simulink model "CV_Matbab_Moteur"  (R2016a)
settings: Solver=FixedStepAuto  StartTime=0.0  StopTime=10  FixedStep=1e-6  RelTol=1e-3
libraries: powerlib x11
settings Model: SimulationMode=accelerator  Creator=SINA  LastModifiedBy=SINA

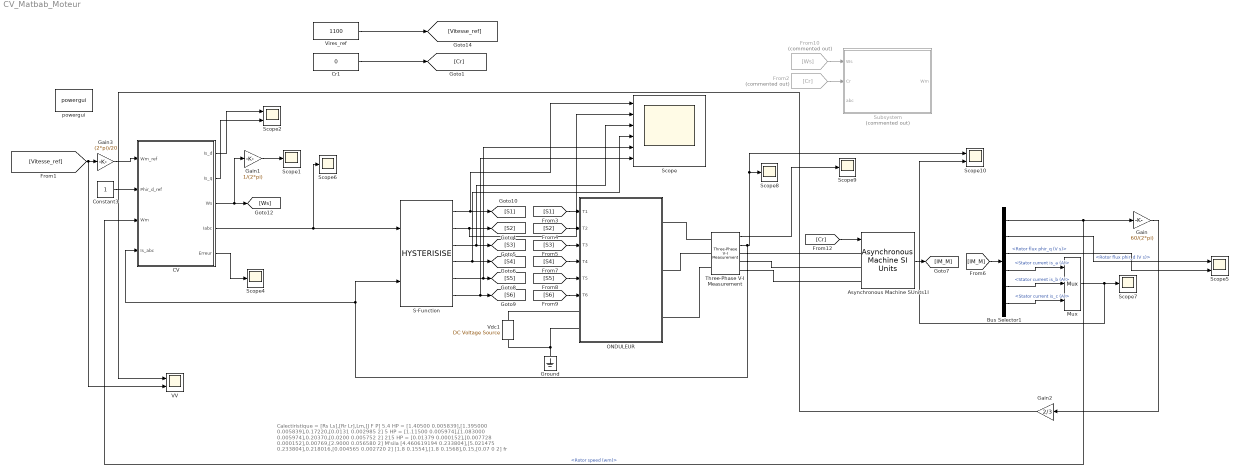
== system CV_Matbab_Moteur ==
  note: Calectiristique = [Rs Ls],[Rr Lr],Lm,[J F P]
      |
      | 5.4 HP = [1.40500 0.005839],[1.395000 0.005839],0.17220,[0.0131 0.002985 2]
      | 5 HP = [1.11500 0.005974],[1.083000 0.005974],0.20370,[0.0200 0.005752 2]
      | 215 HP = [0.01379 0.000152],[0.007728 0.000152],0.00769,[2.9000 0.056580 2]
      |
      | M'sila
      | [4.460619194 0.233804],[5.021475 0.233804],0.218016,[0.004565 0.002720 2]
      |
      | [1.8 0.1554],[1.8 0.1568],0.15,[0.07 0 2] fr
  "Asynchronous Machine SUnits1I " : powerlib/Machines/Asynchronous Machine SI Units  RotorType=Squirrel-cage  PresetModel="15:  5.4 HP (4KW)   400 V  50Hz 1430 RPM"  MechanicalLoad=Torque Tm  ShowDetailedParameters=on  ReferenceFrame=Rotor  Units=SI  MeasurementBus=off  NominalParameters=[4000 400 50]  Stator=[1.405 0.005839]  Rotor=[1.395 0.005839]  Cage1=[0.4155 0.002066]  Cage2=[0.4168 0.0003495]  Lm=0.1722  Mechanical=[0.0131 0.002985 2]  PolePairs=2  InitialConditions=[0 0 0 0 0 0 0 0]  SimulateSaturation=off  Saturation=[14.03593122, 27.81365428, 53.79336849, 72.68890987, 97.98006896, 148.6815601, 215.7428561, 302.9841135, 428.7778367 ; 230, 322, 414, 460, 506, 552, 598, 644, 690]  LoadFlowParameters=1492000  TsPowergui=0  TsBlock=-1  IterativeModel=Trapezoidal non iterative  IterativeDiscreteModel=Trapezoidal non iterative  Pmec=1.492e+006
  Bus Selector1 : BusSelector  OutputSignals=Mechanical.Rotor speed (wm),Rotor measurements.Rotor flux phir_d (V s),Rotor measurements.Rotor flux phir_q (V s),Stator measurements.Stator current is_a (A),Stator measurements.Stator current is_b (A),Stator measurements.Stator current is_c (A)
  CV : Subsystem
  Constant3 : Constant
  Cr1 : Constant  Value=0
  From10 : From  Commented=on  GotoTag=Ws
  From2 : From  Commented=on  GotoTag=Cr
  Gain : Gain  Gain=60/(2*pi)
  Gain1 : Gain  Gain=1/(2*pi)
  Gain2 : Gain  Gain=2/3
  Gain3 : Gain  Gain=(2*pi)/20
  Ground : powerlib/Elements/Ground  LConnTagsString=a
  Mux : Mux  Inputs=3
  ONDULEUR : Subsystem
  S-Function : S-Function  FunctionName=HYSTERISISE  SFunctionDeploymentMode=off  EnableBusSupport=off
  Scope : Scope  NumInputPorts=6
  Scope{1,4,6..9} (6 alike) : Scope
  Scope10 : Scope  NumInputPorts=2
  Scope2 : Scope  NumInputPorts=2
  Scope5 : Scope  NumInputPorts=2
  Subsystem : Subsystem  Commented=on
  Three-Phase V-I Measurement : powerlib/Measurements/Three-Phase V-I Measurement  VoltageMeasurement=phase-to-phase  SetLabelV=off  LabelV=Vabc  Vpu=off  VpuLL=off  CurrentMeasurement=yes  SetLabelI=off  LabelI=Iabc  Ipu=off  Pbase=100e6  Vbase=500e3  OutputType=Complex  PhasorSimulation=off  PSBequivalent=0
  VV : Scope  NumInputPorts=2
  Vdc1 : powerlib/Electrical Sources/DC Voltage Source  Amplitude=650  Measurements=Voltage
  Vires_ref : Constant  Value=1100
  powergui : powerlib/powergui  Priority=1  SimulationMode=Discrete  SolverType=Tustin/Backward Euler (TBE)  SampleTime=1e-6  frequency=60  SPID=off  DisableSnubberDevices=off  DisableRonSwitches=off  DisableVfSwitches=off  SwTol=0  DisplayEquations=off  Interpol=off  ExternalGateDelay=off  methode=off  Ts=0  FunctionMessages=off  echomessages=off  HookPort=off  EnableUseOfTLC=off  x0status=blocks  frequencyindice=0  Pbase=100e6  ErrMax=1e-4  Iterations=50  UnitsV=kV  UnitsW=MW  buscounter=0  RestoreLinks=warning  ResistiveCurrentMeasurement=off  Frange=[0:2:500]  Ylog=off  Xlog=on  ShowGrid=off  save=off  variable=ZData  structure=0  ZoomFFT=on  StartTime=0.0  cycles=1  DisplayStyle=1  fundamental=60  FreqAxis=off  MaxFrequency=1000  frequencyindicesteady=1  RmsSteady=1  display=off
  wires:
  Constant3/1 -> CV/2(Phir_d_ref)
  CV/3(Ws) -> [Ws], Gain1/1
  CV/4(Iabc) -> Scope6/1, S-Function/1
  Gain1/1 -> Scope1/1
  CV/1(Is_d) -> Scope2/1
  CV/2(Is_q) -> Scope2/2
  CV/5(Erreur) -> Scope4/1
  Cr1/1 -> [Cr]
  Vires_ref/1 -> [Vitesse_ref]
  From10/1 -> Subsystem/1(Ws)
  From2/1 -> Subsystem/2(Cr)
  [IM_M] -> Bus Selector1/1
  Bus Selector1/1 -> CV/3(Wm), Gain/1  "<Rotor speed (wm)>"
  "Asynchronous Machine SUnits1I "/1 -> [IM_M]
  [Cr] -> "Asynchronous Machine SUnits1I "/1
  Bus Selector1/2 -> Scope5/1  "<Rotor flux phir_d (V s)>"
  Bus Selector1/3 -> Scope5/2  "<Rotor flux phir_q (V s)>"
  [S1] -> ONDULEUR/1("T1 ")
  [S3] -> ONDULEUR/3("T3  ")
  [S5] -> ONDULEUR/5("T5 ")
  [S2] -> ONDULEUR/2("T2 ")
  [S4] -> ONDULEUR/4("T4 ")
  [S6] -> ONDULEUR/6("T6 ")
  S-Function/5 -> Scope/5, [S5]
  S-Function/4 -> Scope/4, [S4]
  S-Function/3 -> Scope/3, [S3]
  S-Function/2 -> Scope/2, [S2]
  S-Function/1 -> Scope/1, [S1]
  Bus Selector1/4 -> Mux/1  "<Stator current is_a (A)>"
  Bus Selector1/5 -> Mux/2  "<Stator current is_b (A)>"
  Bus Selector1/6 -> Mux/3  "<Stator current is_c (A)>"
  Mux/1 -> Scope10/2, Scope7/1
  S-Function/6 -> Scope/6, [S6]
  Three-Phase V-I Measurement/2 -> S-Function/2, CV/4(Is_abc), Scope10/1, Scope8/1
  Three-Phase V-I Measurement/1 -> Scope9/1
  [Vitesse_ref] -> VV/2, Gain3/1
  Gain3/1 -> CV/1(Wm_ref)
  Gain/1 -> Gain2/1
  Gain2/1 -> VV/1
  connections:
  Three-Phase V-I Measurement/LConn3 -- ONDULEUR/RConn3
  Three-Phase V-I Measurement/LConn2 -- ONDULEUR/RConn2
  Three-Phase V-I Measurement/LConn1 -- ONDULEUR/RConn1
  Three-Phase V-I Measurement/RConn1 -- "Asynchronous Machine SUnits1I "/LConn1
  Three-Phase V-I Measurement/RConn2 -- "Asynchronous Machine SUnits1I "/LConn2
  Three-Phase V-I Measurement/RConn3 -- "Asynchronous Machine SUnits1I "/LConn3
  Vdc1/RConn1 -- ONDULEUR/LConn1
  Ground/LConn1 -- ONDULEUR/LConn2 -- Vdc1/LConn1

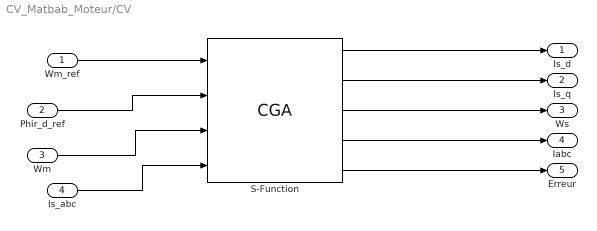
== system CV_Matbab_Moteur/CV ==
  Wm_ref : Inport
  Phir_d_ref : Inport  Port=2
  Wm : Inport  Port=3
  Is_abc : Inport  Port=4
  S-Function : S-Function  FunctionName=CGA  Parameters=[1.40500 0.005839],[1.395000 0.005839],0.17220,[0.0131 0.002985 2]  SFunctionDeploymentMode=off  EnableBusSupport=off
  Is_d : Outport
  Is_q : Outport  Port=2
  Ws : Outport  Port=3
  Iabc : Outport  Port=4
  Erreur : Outport  Port=5
  wires:
  S-Function/4 -> Iabc/1
  S-Function/3 -> Ws/1
  S-Function/2 -> Is_q/1
  S-Function/1 -> Is_d/1
  Wm/1 -> S-Function/3
  Phir_d_ref/1 -> S-Function/2
  Wm_ref/1 -> S-Function/1
  S-Function/5 -> Erreur/1
  Is_abc/1 -> S-Function/4

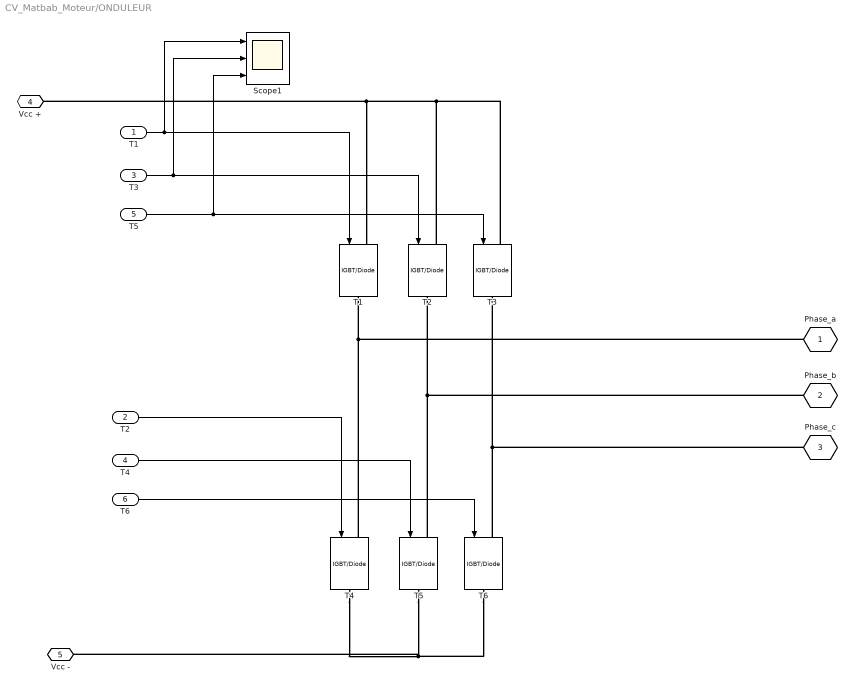
== system CV_Matbab_Moteur/ONDULEUR ==
  "T1 " : Inport
  "T2 " : Inport  Port=2
  "T3  " : Inport  Port=3
  "T4 " : Inport  Port=4
  "T5 " : Inport  Port=5
  "T6 " : Inport  Port=6
  Scope1 : Scope  NumInputPorts=3
  T{1..6} (6 alike) : powerlib/Power Electronics/IGBT//Diode  Ron=1e-3  Rs=1e5  Cs=inf  Measurements=off
  Phase_a : PMIOPort  Tag=PMCPort  Port=1  Side=Right
  Phase_b : PMIOPort  Tag=PMCPort  Port=2  Side=Right
  Phase_c : PMIOPort  Tag=PMCPort  Port=3  Side=Right
  Vcc + : PMIOPort  Port=4  Side=Left
  Vcc - : PMIOPort  Port=5  Side=Left
  wires:
  "T1 "/1 -> Scope1/1, T1/1
  "T3  "/1 -> Scope1/2, T2/1
  "T5 "/1 -> Scope1/3, T3/1
  "T2 "/1 -> T4/1
  "T4 "/1 -> T5/1
  "T6 "/1 -> T6/1
  connections:
  T2/LConn1 -- T3/LConn1 -- Vcc +/RConn1 -- T1/LConn1
  T5/RConn1 -- T4/RConn1 -- Vcc -/RConn1 -- T6/RConn1
  T4/LConn1 -- Phase_a/RConn1 -- T1/RConn1
  T5/LConn1 -- Phase_b/RConn1 -- T2/RConn1
  T6/LConn1 -- Phase_c/RConn1 -- T3/RConn1

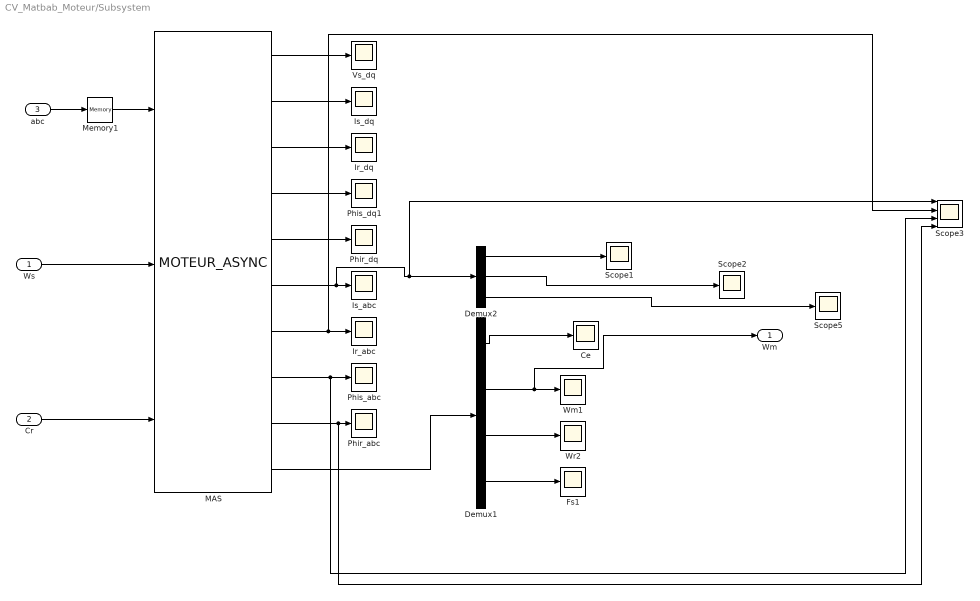
== system CV_Matbab_Moteur/Subsystem ==
  Ws : Inport
  Cr : Inport  Port=2
  abc : Inport  Port=3
  Ce : Scope
  Demux1 : Demux
  Demux2 : Demux  Outputs=3
  Fs1 : Scope
  Ir_abc : Scope
  Ir_dq : Scope
  Is_abc : Scope
  Is_dq : Scope
  MAS : S-Function  FunctionName=MOTEUR_ASYNC  Parameters=[1.40500 0.005839],[1.395000 0.005839],0.17220,[0.0131 0.002985 2]  SFunctionDeploymentMode=off  EnableBusSupport=off
  Memory1 : Memory
  Phir_abc : Scope
  Phir_dq : Scope
  Phis_abc : Scope
  Phis_dq1 : Scope
  Scope1 : Scope
  Scope2 : Scope
  Scope3 : Scope  NumInputPorts=4
  Scope5 : Scope
  Vs_dq : Scope
  Wm1 : Scope
  Wr2 : Scope
  Wm : Outport
  wires:
  Demux2/3 -> Scope5/1
  Demux1/2 -> Wm/1, Wm1/1
  Demux1/3 -> Wr2/1
  Ws/1 -> MAS/2
  MAS/7 -> Scope3/2, Ir_abc/1
  MAS/9 -> Scope3/4, Phir_abc/1
  MAS/2 -> Is_dq/1
  Demux1/4 -> Fs1/1
  MAS/6 -> Scope3/1, Demux2/1, Is_abc/1
  Demux1/1 -> Ce/1
  MAS/5 -> Phir_dq/1
  MAS/10 -> Demux1/1
  MAS/8 -> Scope3/3, Phis_abc/1
  MAS/4 -> Phis_dq1/1
  MAS/1 -> Vs_dq/1
  Cr/1 -> MAS/3
  MAS/3 -> Ir_dq/1
  Demux2/1 -> Scope1/1
  Demux2/2 -> Scope2/1
  Memory1/1 -> MAS/1
  abc/1 -> Memory1/1
